simulink model "Single_Axis_Roll_Disturbance"  (R2024b)
settings: Solver=ode4  StartTime=0.0  StopTime=0.2  FixedStep=0.001  RelTol=1e-3
settings Model: Creator=Zohaib  LastModifiedBy=Zohaib
settings DataIOCC: ReturnWorkspaceOutputs=off

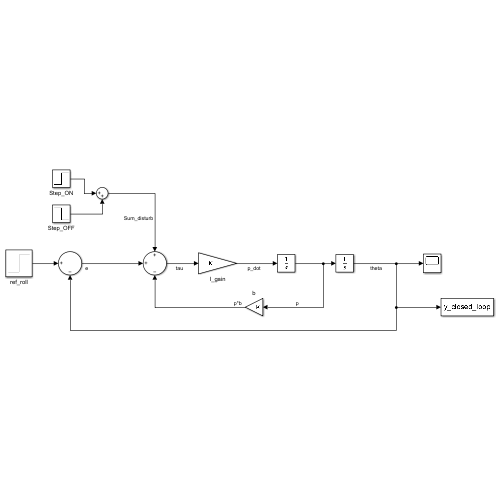
[thumbnail: Simulink's stored preview of the top-level diagram]
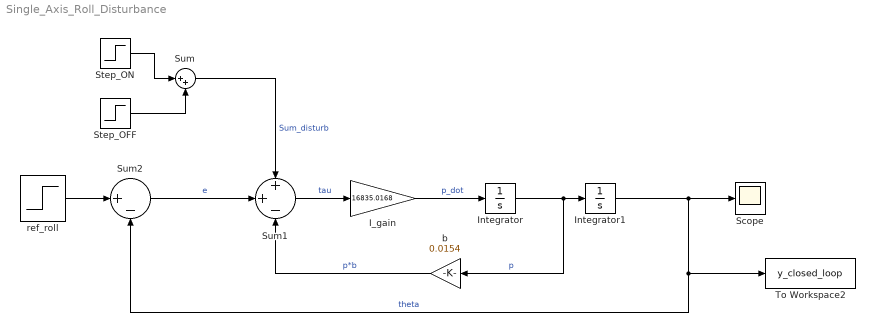
== system Single_Axis_Roll_Disturbance ==
  I_gain : Gain  Gain=16835.0168
  Integrator : Integrator
  Integrator1 : Integrator
  Scope : Scope
  Step_OFF : Step  Time=0.105  After=-0.015  SampleTime=0.001
  Step_ON : Step  Time=0.1  After=0.015  SampleTime=0.001
  Sum : Sum  Inputs=|++
  Sum1 : Sum  Inputs=++-
  Sum2 : Sum  Inputs=|+-
  To Workspace2 : ToWorkspace  VariableName=y_closed_loop  SaveFormat=Timeseries  SampleTime=-1
  b : Gain  Gain=0.0154
  ref_roll : Step  Time=0  After=5*(pi/180)  SampleTime=0.001
  wires:
  Integrator1/1 -> To Workspace2/1, Sum2/2, Scope/1  "theta"
  Integrator/1 -> b/1, Integrator1/1  "p"
  I_gain/1 -> Integrator/1  "p_dot"
  Sum1/1 -> I_gain/1  "tau"
  ref_roll/1 -> Sum2/1
  Step_ON/1 -> Sum/1
  Step_OFF/1 -> Sum/2
  b/1 -> Sum1/3  "p*b"
  Sum2/1 -> Sum1/2  "e"
  Sum/1 -> Sum1/1  "Sum_disturb"
